simulink model "RobotX_AcousticPoint"  (R2014a)
settings: Solver=FixedStepDiscrete  StartTime=0.0  StopTime=inf  FixedStep=.25  RelTol=1e-3
undefined symbols (not defined in the file): Com1, Com2, Com3, Com4, DiscIntNeverNeededParam, standard
libraries: xpcseriallib x11, simulink x7, slrtlib x5, speedgoatlib x1, speedgoatlib_IO102 x1
(part 2 of 2)

== matlab function RobotX_AcousticPoint/Main FSM/Acoustic FSM/Drive Pt2/CalcTimes ==
  data: pts input; u input; Data output
function Data = calcTimes(pts, u)
%Written by Anderson Lebbad on August 9, 2014
%Last Edited: Dylan DeGaetano September 1, 2014

%Calculates times for the boat to get to points for a trajectory, and
%formats Data for communication

%Initialize
Data = zeros(24,1);
traj = zeros(8,3);
traj(:,1:2) = pts;



for k = 2:8
    %Calculate distance to travel from last point
    distTravel = sqrt(sum((pts(k-1,:)-pts(k,:)).^2));
    %Assume 1m per second speed
    traj(k,3) = traj(k-1,3) + distTravel;
    %Add time based off initial velocity to get to first point past initial
    if k == 2
        traj(k,3) = traj(k,3) + 2.5*abs(2-u);
    end
end


%Output Data
for i=1:8
    for j = 1:3
        Data(3*(i-1)+j) = traj(i,j);
    end
end

== matlab function RobotX_AcousticPoint/Main FSM/Acoustic FSM/Drive Pt1/GPSMove ==
  data: X input; Finished output; valid output; Y input; Psi input; Targets input; pts output
function [Finished, valid, pts] = GPSmove(X,Y,Psi,Targets)
%Written by Dylan DeGaetano on September 1, 2014
%Last edited by: Michael Benson on September 4, 2014
%   Changed Sample to be a persistent variable so that pts will not be
%   recalculated every iteration.
%
%This function will go to a given NED cooridnate 

GoalPt = Targets(1,:);

persistent Sample

if isempty(Sample)
    Sample = 0;
end

valid = 0;
Finished = 0;
pts = zeros(8,2);
%$Distance to object in meters

if Sample == 0
    valid = 1;
    pts(1,1) = X+5*cos(Psi*pi/180);
    pts(1,2) = Y+5*cos(Psi*pi/180);
    pts(8,1) = GoalPt(1,1);
    pts(8,2) = GoalPt(1,2);
    pts(2,:) = pts(1,:) +(1*(GoalPt-pts(1,:))/7);
    pts(3,:) = pts(1,:) +(2*(GoalPt-pts(1,:))/7);
    pts(4,:) = pts(1,:) +(3*(GoalPt-pts(1,:))/7);
    pts(5,:) = pts(1,:) +(4*(GoalPt-pts(1,:))/7);
    pts(6,:) = pts(1,:) +(5*(GoalPt-pts(1,:))/7);
    pts(7,:) = pts(1,:) +(6*(GoalPt-pts(1,:))/7);
    Sample = 1; 
else 
    range = sqrt(sum((GoalPt - [X Y]).^2));
    if range <= 3
        Finished = 1;
    end
end

== matlab function RobotX_AcousticPoint/Main FSM/Acoustic FSM/Drive Pt2/GPSMove ==
  data: X input; Finished output; valid output; Y input; Psi input; Targets input; pts output
function [Finished, valid, pts] = GPSmove(X,Y,Psi,Targets)
%Written by Dylan DeGaetano on September 1, 2014
%Last edited by: Michael Benson on September 4, 2014
%   Changed Sample to be a persistent variable so that pts will not be
%   recalculated every iteration.
%
%This function will go to a given NED cooridnate 

GoalPt = Targets(2,:);

persistent Sample

if isempty(Sample)
    Sample = 0;
end

valid = 0;
Finished = 0;
pts = zeros(8,2);
%$Distance to object in meters

if Sample == 0
    valid = 1;
    pts(1,1) = X+5*cos(Psi*pi/180);
    pts(1,2) = Y+5*cos(Psi*pi/180);
    pts(8,1) = GoalPt(1,1);
    pts(8,2) = GoalPt(1,2);
    pts(2,:) = pts(1,:) +(1*(GoalPt-pts(1,:))/7);
    pts(3,:) = pts(1,:) +(2*(GoalPt-pts(1,:))/7);
    pts(4,:) = pts(1,:) +(3*(GoalPt-pts(1,:))/7);
    pts(5,:) = pts(1,:) +(4*(GoalPt-pts(1,:))/7);
    pts(6,:) = pts(1,:) +(5*(GoalPt-pts(1,:))/7);
    pts(7,:) = pts(1,:) +(6*(GoalPt-pts(1,:))/7);
    Sample = 1; 
else 
    range = sqrt(sum((GoalPt - [X Y]).^2));
    if range <= 3
        Finished = 1;
    end
end

== matlab function RobotX_AcousticPoint/Main FSM/Acoustic FSM/Drive Pt3/CalcTimes ==
  data: pts input; u input; Data output
function Data = calcTimes(pts, u)
%Written by Anderson Lebbad on August 9, 2014
%Last Edited: Dylan DeGaetano September 1, 2014

%Calculates times for the boat to get to points for a trajectory, and
%formats Data for communication

%Initialize
Data = zeros(24,1);
traj = zeros(8,3);
traj(:,1:2) = pts;



for k = 2:8
    %Calculate distance to travel from last point
    distTravel = sqrt(sum((pts(k-1,:)-pts(k,:)).^2));
    %Assume 1m per second speed
    traj(k,3) = traj(k-1,3) + distTravel;
    %Add time based off initial velocity to get to first point past initial
    if k == 2
        traj(k,3) = traj(k,3) + 2.5*abs(2-u);
    end
end


%Output Data
for i=1:8
    for j = 1:3
        Data(3*(i-1)+j) = traj(i,j);
    end
end

== matlab function RobotX_AcousticPoint/Main FSM/Acoustic FSM/Point/Point ==
  data: AcousticPose1 input; AcousticPose2 input; AcousticPose3 input; Data output; X input; Y input
function Data  = PingPoint(AcousticPose1,AcousticPose2,AcousticPose3,X,Y)
%Written by Anderson Lebbad on September 13, 2014
%Last Edited:

%This function causes the vessel point at the estimated location of the
%pinger

%% Calculate the NED point by finding the three intersections and averaging

%First intersection
compMat = [cos(AcousticPose1(3)), sin(AcousticPose1(3)); cos(AcousticPose2(3)), sin(AcousticPose2(3))];
intScales = [(AcousticPose2(1)-AcousticPose1(1)), (AcousticPose2(2)-AcousticPose1(2))]/compMat;
pingPose1 = [(AcousticPose1(1)+intScales(1)*compMat(1,1)), (AcousticPose1(2)+intScales(1)*compMat(1,2))];

%Second intersection
compMat = [cos(AcousticPose1(3)), sin(AcousticPose1(3)); cos(AcousticPose3(3)), sin(AcousticPose3(3))];
intScales = [(AcousticPose3(1)-AcousticPose1(1)), (AcousticPose3(2)-AcousticPose1(2))]/compMat;
pingPose2 = [(AcousticPose1(1)+intScales(1)*compMat(1,1)), (AcousticPose1(2)+intScales(1)*compMat(1,2))];

%Second intersection
compMat = [cos(AcousticPose2(3)) sin(AcousticPose2(3)); cos(AcousticPose3(3)) sin(AcousticPose3(3))];
intScales = [(AcousticPose3(1)-AcousticPose2(1)), (AcousticPose3(2)-AcousticPose2(2))]/compMat;
pingPose3 = [(AcousticPose2(1)+intScales(1)*compMat(1,1)), (AcousticPose2(2)+intScales(1)*compMat(1,2))];

PingPose = (pingPose1+pingPose2+pingPose3)/3;

%% Point at the pose
Theta = atan2(PingPose(2)-Y,PingPose(1)-X);
Data = zeros(24,1);
Data(1) = X;
Data(2) = Y;
Data(3) = Theta*180/pi;


end

== matlab function RobotX_AcousticPoint/Main FSM/Acoustic FSM/Acoustics Pt1/Ping Point ==
  data: Deployed input; finished output; X input; Y input; Psi input; HorizBearing input; NewBearing input; Data output; acousticPose output
function [finished,Data,acousticPose] = PingPoint(Deployed,X,Y,Psi,HorizBearing,NewBearing)
%Written by Anderson Lebbad on September 12, 2014
%Last Edited:

%This function causes the vessel to spin in place until a ping is detected,
%then orients itself towards the direction of the source of that ping

persistent holdPose Pinged aveHeading aveXY

if isempty(holdPose)
    holdPose = [X Y Psi];
    Pinged = 0;
    aveHeading = [0 0]; %Two elements, first is running average, second is accumulator
    aveXY = [0 0]; %Two elements, X ave and Y ave
end

%Initialize output variables
finished = 0;
Data = zeros(24,1);


%Angular offset (indirect rate control)
offset = 5;

%Only move once flagged as deployed
if Deployed == 1
    %If it hasn't heard a ping yet, spin
    if Pinged == 0
        holdPose(3) = mod(Psi + offset,360);
    end
    
    %If the ping is less than 250 milliseconds (a timestep) then point at the
    %direction of sound
    if abs(HorizBearing) >= 15
        if NewBearing
            holdPose(3) = mod(Psi + HorizBearing,360);
            Pinged = 1;
        end
    end
    
    %If it gets a new acoustic sample, increment the running average
    if NewBearing
        aveHeading(2) = aveHeading(2) + 1;
        aveHeading(1) = (aveHeading(1)*(aveHeading(2)-1)+(Psi+HorizBearing))/aveHeading(2);
        %In case of drift, keep a running average of the XY coordinates as well
        aveXY(1) = (aveXY(1)*(aveHeading(2)-1)+X)/aveHeading(2);
        aveXY(2) = (aveXY(2)*(aveHeading(2)-1)+Y)/aveHeading(2);
    end
    
    if aveHeading(2) >= 16
        finished = 1;
    end
end

%Set desired pose
Data(1) = holdPose(1);
Data(2) = holdPose(2);
Data(3) = holdPose(3);

acousticPose = [aveXY aveHeading(1)];

== matlab function RobotX_AcousticPoint/Main FSM/Acoustic FSM/Drive Pt3/GPSMove ==
  data: X input; Finished output; valid output; Y input; Psi input; Targets input; pts output
function [Finished, valid, pts] = GPSmove(X,Y,Psi,Targets)
%Written by Dylan DeGaetano on September 1, 2014
%Last edited by: Michael Benson on September 4, 2014
%   Changed Sample to be a persistent variable so that pts will not be
%   recalculated every iteration.
%
%This function will go to a given NED cooridnate 

GoalPt = Targets(3,:);

persistent Sample

if isempty(Sample)
    Sample = 0;
end

valid = 0;
Finished = 0;
pts = zeros(8,2);
%$Distance to object in meters

if Sample == 0
    valid = 1;
    pts(1,1) = X+5*cos(Psi*pi/180);
    pts(1,2) = Y+5*cos(Psi*pi/180);
    pts(8,1) = GoalPt(1,1);
    pts(8,2) = GoalPt(1,2);
    pts(2,:) = pts(1,:) +(1*(GoalPt-pts(1,:))/7);
    pts(3,:) = pts(1,:) +(2*(GoalPt-pts(1,:))/7);
    pts(4,:) = pts(1,:) +(3*(GoalPt-pts(1,:))/7);
    pts(5,:) = pts(1,:) +(4*(GoalPt-pts(1,:))/7);
    pts(6,:) = pts(1,:) +(5*(GoalPt-pts(1,:))/7);
    pts(7,:) = pts(1,:) +(6*(GoalPt-pts(1,:))/7);
    Sample = 1; 
else 
    range = sqrt(sum((GoalPt - [X Y]).^2));
    if range <= 3
        Finished = 1;
    end
end

== matlab function RobotX_AcousticPoint/Main FSM/Acoustic FSM/Acoustics Pt2/Ping Point ==
  data: Deployed input; finished output; X input; Y input; Psi input; HorizBearing input; NewBearing input; Data output; acousticPose output
function [finished,Data,acousticPose] = PingPoint(Deployed,X,Y,Psi,HorizBearing,NewBearing)
%Written by Anderson Lebbad on September 12, 2014
%Last Edited:

%This function causes the vessel to spin in place until a ping is detected,
%then orients itself towards the direction of the source of that ping

persistent holdPose Pinged aveHeading aveXY

if isempty(holdPose)
    holdPose = [X Y Psi];
    Pinged = 0;
    aveHeading = [0 0]; %Two elements, first is running average, second is accumulator
    aveXY = [0 0]; %Two elements, X ave and Y ave
end

%Initialize output variables
finished = 0;
Data = zeros(24,1);


%Angular offset (indirect rate control)
offset = 5;

%Only move once flagged as deployed
if Deployed == 1
    %If it hasn't heard a ping yet, spin
    if Pinged == 0
        holdPose(3) = mod(Psi + offset,360);
    end
    
    %If the ping is less than 250 milliseconds (a timestep) then point at the
    %direction of sound
    if abs(HorizBearing) >= 15
        if NewBearing
            holdPose(3) = mod(Psi + HorizBearing,360);
            Pinged = 1;
        end
    end
    
    %If it gets a new acoustic sample, increment the running average
    if NewBearing
        aveHeading(2) = aveHeading(2) + 1;
        aveHeading(1) = (aveHeading(1)*(aveHeading(2)-1)+(Psi+HorizBearing))/aveHeading(2);
        %In case of drift, keep a running average of the XY coordinates as well
        aveXY(1) = (aveXY(1)*(aveHeading(2)-1)+X)/aveHeading(2);
        aveXY(2) = (aveXY(2)*(aveHeading(2)-1)+Y)/aveHeading(2);
    end
    
    if aveHeading(2) >= 16
        finished = 1;
    end
end

%Set desired pose
Data(1) = holdPose(1);
Data(2) = holdPose(2);
Data(3) = holdPose(3);

acousticPose = [aveXY aveHeading(1)];

== matlab function RobotX_AcousticPoint/Main FSM/Acoustic FSM/Acoustics Pt3/Ping Point ==
  data: Deployed input; finished output; X input; Y input; Psi input; HorizBearing input; NewBearing input; Data output; acousticPose output
function [finished,Data,acousticPose] = PingPoint(Deployed,X,Y,Psi,HorizBearing,NewBearing)
%Written by Anderson Lebbad on September 12, 2014
%Last Edited:

%This function causes the vessel to spin in place until a ping is detected,
%then orients itself towards the direction of the source of that ping

persistent holdPose Pinged aveHeading aveXY

if isempty(holdPose)
    holdPose = [X Y Psi];
    Pinged = 0;
    aveHeading = [0 0]; %Two elements, first is running average, second is accumulator
    aveXY = [0 0]; %Two elements, X ave and Y ave
end

%Initialize output variables
finished = 0;
Data = zeros(24,1);


%Angular offset (indirect rate control)
offset = 5;

%Only move once flagged as deployed
if Deployed == 1
    %If it hasn't heard a ping yet, spin
    if Pinged == 0
        holdPose(3) = mod(Psi + offset,360);
    end
    
    %If the ping is less than 250 milliseconds (a timestep) then point at the
    %direction of sound
    if abs(HorizBearing) >= 15
        if NewBearing
            holdPose(3) = mod(Psi + HorizBearing,360);
            Pinged = 1;
        end
    end
    
    %If it gets a new acoustic sample, increment the running average
    if NewBearing
        aveHeading(2) = aveHeading(2) + 1;
        aveHeading(1) = (aveHeading(1)*(aveHeading(2)-1)+(Psi+HorizBearing))/aveHeading(2);
        %In case of drift, keep a running average of the XY coordinates as well
        aveXY(1) = (aveXY(1)*(aveHeading(2)-1)+X)/aveHeading(2);
        aveXY(2) = (aveXY(2)*(aveHeading(2)-1)+Y)/aveHeading(2);
    end
    
    if aveHeading(2) >= 16
        finished = 1;
    end
end

%Set desired pose
Data(1) = holdPose(1);
Data(2) = holdPose(2);
Data(3) = holdPose(3);

acousticPose = [aveXY aveHeading(1)];

== matlab function RobotX_AcousticPoint/Main FSM/Main Enabler ==
  data: taskSelector output; initEn output; acousticEn output; RCEn output; OnOffRCAuto input; initFin input
function [taskSelector,initEn,acousticEn,RCEn] = taskEnabler(OnOffRCAuto, initFin)
%Written by Anderson Lebbad on September 13, 2014
%Last Edited by:

%Changes the value of MainMode and the enablers for the tasks within the
%Main FSM.

% Initialize enable signals
RCEn = 0;
initEn = 0;
acousticEn = 0;

% Set enable signals based on state completion
if initFin == 0
    initEn = 1;
    taskSelector = 1;
elseif OnOffRCAuto ~= 3
    RCEn = 1;
    taskSelector = 3;
else
    acousticEn = 1;
    taskSelector = 2;
end

== matlab function RobotX_AcousticPoint/Main FSM/RCHold/Set Pose ==
  data: X input; Data output; Y input; Psi input
function Data = setPose(X,Y,Psi)
%Written by Anderson Lebbad on August 9, 2014
%Last Edited:

%This function passes the current pose data with a heading offset as the
%desired pose for the station keeping controller to use.

persistent holdPose

if isempty(holdPose)
    holdPose = [X Y Psi];
end

%Initialize Data variable
Data = zeros(24,1);

%Set desired pose
Data(1) = holdPose(1);
Data(2) = holdPose(2);
Data(3) = holdPose(3);
